simulink model "Stage_2_1_Virtual_CAN_Network"  (R2025a)
settings: Solver=VariableStepAuto  StartTime=0.0  StopTime=10.0  RelTol=1e-3
libraries: canmsglib x2
settings Model: Creator=sitam  LastModifiedBy=sitam

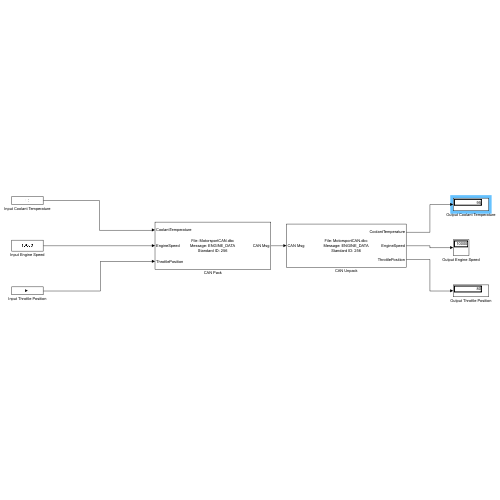
[thumbnail: Simulink's stored preview of the top-level diagram]
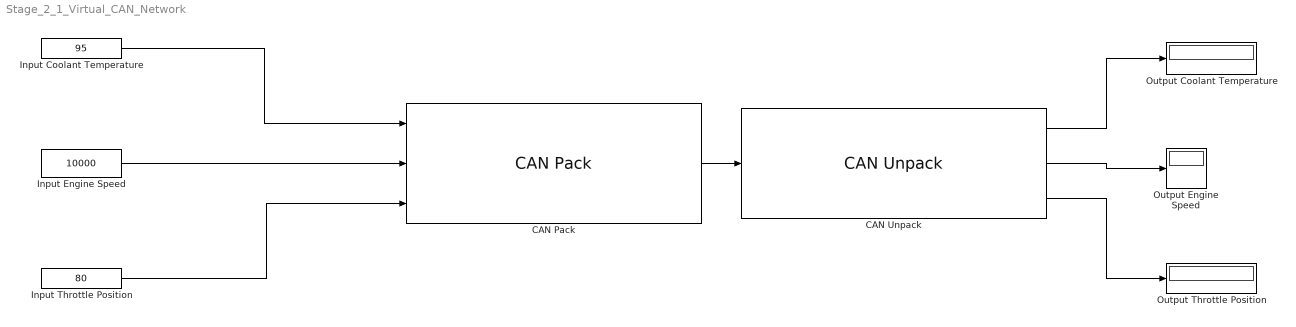
== system Stage_2_1_Virtual_CAN_Network ==
  CAN Pack : canmsglib/CAN Pack  CANdbFile=C:\Users\sitam\OneDrive\Projects\CAN Bus Project\MotorsportCAN.dbc  MsgList=ENGINE_DATA  MsgName=ENGINE_DATA  MsgIDType=Standard (11-bit identifier)  MsgIdentifier=256  CANIDInput=off  MsgLength=8  Remote=off  ApplyMinMax=off  BusOutput=off  SignalInfo={'CoolantTemperature','24','8','LE','unsigned','Standard','0','1','-40','-40','150';'EngineSpeed','0','16','LE','unsigned','Standard','0','0.25','0','0','15000';'ThrottlePosition','16','8','LE','unsigned','Standard','0','0.4','0','0','100'}
      settings: LibrarySourceBlock=canlib/CAN Pack  DataFormat=CANdb specified signals
  CAN Unpack : canmsglib/CAN Unpack  CANdbFile=C:\Users\sitam\OneDrive\Projects\CAN Bus Project\MotorsportCAN.dbc  MsgList=ENGINE_DATA  MsgName=ENGINE_DATA  MsgIDType=Standard (11-bit identifier)  MsgIdentifier=256  MsgLength=8  SignalInfo={'CoolantTemperature','24','8','LE','unsigned','Standard','0','1','-40','-40','150';'EngineSpeed','0','16','LE','unsigned','Standard','0','0.25','0','0','15000';'ThrottlePosition','16','8','LE','unsigned','Standard','0','0.4','0','0','100'}  IDPort=off  TimestampPort=off  ErrorPort=off  RemotePort=off  LengthPort=off  StatusPort=off  ApplyMinMax=off
      settings: LibrarySourceBlock=canlib/CAN Unpack  DataFormat=CANdb specified signals
  Input Coolant Temperature : Constant  Value=95
  Input Engine Speed : Constant  Value=10000
  Input Throttle Position : Constant  Value=80
  Output Coolant Temperature : Display
  Output Engine Speed : Display
  Output Throttle Position : Display
  wires:
  CAN Pack/1 -> CAN Unpack/1
  Input Engine Speed/1 -> CAN Pack/2
  Input Throttle Position/1 -> CAN Pack/3
  Input Coolant Temperature/1 -> CAN Pack/1
  CAN Unpack/2 -> Output Engine Speed/1
  CAN Unpack/1 -> Output Coolant Temperature/1
  CAN Unpack/3 -> Output Throttle Position/1
